simulink model "sim_kuka_model_ik"  (R2021a)
settings: Solver=VariableStepAuto  StartTime=0.0  StopTime=10.0  RelTol=1e-3
undefined symbols (not defined in the file): dhParametersStruct, q1, q2, q3, q4, q5, q6, TT
libraries: lib_Solver x1
settings Model: Creator=chiar  LastModifiedBy=chiar

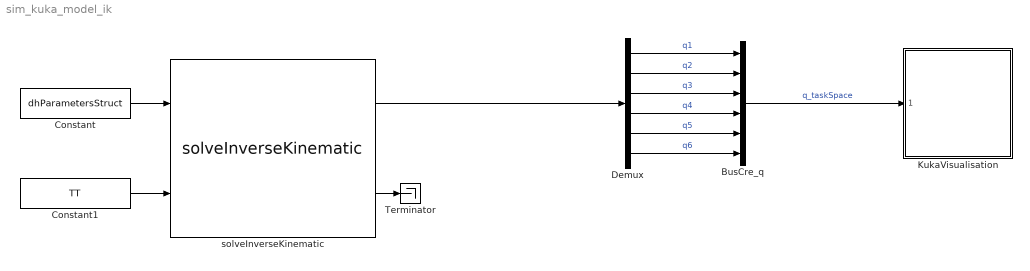
== system sim_kuka_model_ik ==
  BusCre_q : BusCreator  Inputs=q1,q2,q3,q4,q5,q6  OutDataTypeStr=Bus: Bus_q
  Constant : Constant  Value=dhParametersStruct  OutDataTypeStr=Bus: Bus_dhParameter
  Constant1 : Constant  Value=TT
  Demux : Demux  Outputs=6
  KukaVisualisation : Subsystem  ReferencedSubsystem=KukaVisualisationModel
  Terminator : Terminator
  solveInverseKinematic : lib_Solver/solveInverseKinematic  SystemSampleTime=-1  VariantActivationTime=update diagram  Latency=0  AutoFrameSizeCalculation=off
  wires:
  Demux/4 -> BusCre_q/4  "q4"
  solveInverseKinematic/1 -> Demux/1
  Demux/3 -> BusCre_q/3  "q3"
  Constant1/1 -> solveInverseKinematic/2
  Constant/1 -> solveInverseKinematic/1
  solveInverseKinematic/2 -> Terminator/1
  Demux/1 -> BusCre_q/1  "q1"
  Demux/2 -> BusCre_q/2  "q2"
  Demux/6 -> BusCre_q/6  "q6"
  Demux/5 -> BusCre_q/5  "q5"
  BusCre_q/1 -> KukaVisualisation/1  "q_taskSpace"
